simulink model "Starting_v2"  (R2020b)
settings: Solver=ode45  StartTime=0.0  StopTime=0.6  MaxStep=1e-6  RelTol=1e-3
InitFcn:
  | Parameters
undefined symbols (not defined in the file): C_LUT, E_in, fsw, Io_target, ki, kp, L_in, R_in, R_LUT, R_sd, V_OC_LUT, V_soc_0
libraries: simulink x3
settings Model: Creator=sandr  LastModifiedBy=sandr

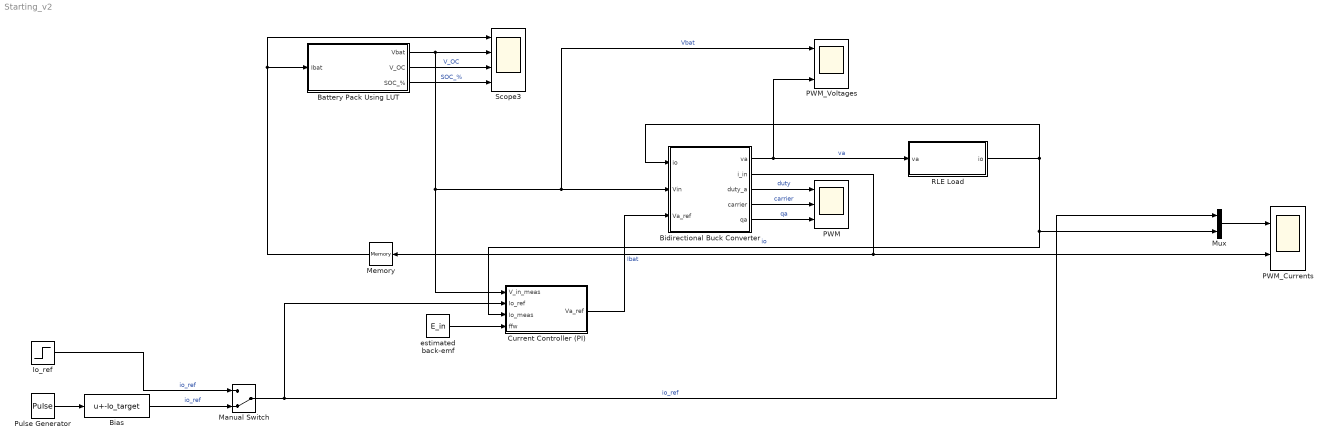
== system Starting_v2 ==
  Battery Pack Using LUT : Subsystem  mask(Battery Pack Model){Cq=C_LUT, Rsd=R_sd, V_SOC_0=V_soc_0, data=V_OC_LUT, R0=R_LUT}
      mask prompts: Cq "Battery Capacity - Cq (As)"; Rsd "Internal Discharging Resistance - Rsd (Ohm)"; V_SOC_0 "Initial V_SOC_0"; data "V_OC from LUT"; R0 "Series Resistance - R0 (Ohm)"
      mask help: This block implements the model of a battery pack.
      mask Help: Author: Sandro Rubino
  Bias : Bias  Bias=-Io_target
  Bidirectional Buck Converter : Subsystem  mask(Bidirectional Buck Converter){fsw=fsw}
      mask prompts: fsw "Switching Frequency - fsw (Hz)"
  Current Controller (PI) : Subsystem  mask(Current Controller (PI Regulator)){kp=kp, ki=ki}
      mask prompts: kp "Proportional Gain - kp (V/A)"; ki "Integral Gain - ki (V/A/s)"
      mask help: This block implments a PI regulator/controller for current control.
  Io_ref : Step  Time=0.3  After=800  SampleTime=0
  Manual Switch : ManualSwitch  CurrentSetting=0
  Memory : Memory
  Mux : Mux  Inputs=2
  PWM : Scope  NumInputPorts=3
  PWM_Currents : Scope  NumInputPorts=2
  PWM_Voltages : Scope  NumInputPorts=3
  Pulse Generator : DiscretePulseGenerator  PulseType=Time based  Amplitude=2*Io_target  Period=0.2  PulseWidth=50
  RLE Load : Subsystem  mask(RLE Load){R=R_in, L=L_in, E=E_in}
      mask prompts: R "Resistance - R (ohm)"; L "Inductance - L (H)"; E "Back-emf - E (V)"
  Scope3 : Scope  NumInputPorts=4
  estimated back-emf : Constant  Value=E_in
  wires:
  Battery Pack Using LUT/3(SOC_%) -> Scope3/4  "SOC_%"
  Battery Pack Using LUT/2(V_OC) -> Scope3/3  "V_OC"
  Battery Pack Using LUT/1(Vbat) -> Current Controller (PI)/1(V_in_meas), PWM_Voltages/1, Bidirectional Buck Converter/2(Vin), Scope3/2  "Vbat"
  Bidirectional Buck Converter/1(va) -> PWM_Voltages/3, RLE Load/1(va)  "va"
  RLE Load/1(io) -> Current Controller (PI)/3(Io_meas), Mux/2, Bidirectional Buck Converter/1(io)  "io"
  Bidirectional Buck Converter/2(i_in) -> Memory/1, PWM_Currents/2  "Ibat"
  Memory/1 -> Battery Pack Using LUT/1(Ibat), Scope3/1
  Bidirectional Buck Converter/3(duty_a) -> PWM/1  "duty"
  Bidirectional Buck Converter/4(carrier) -> PWM/2  "carrier"
  Bidirectional Buck Converter/5(qa) -> PWM/3  "qa"
  Mux/1 -> PWM_Currents/1
  Current Controller (PI)/1(Va_ref) -> Bidirectional Buck Converter/3(Va_ref)
  Manual Switch/1 -> Current Controller (PI)/2(Io_ref), Mux/1  "io_ref"
  Pulse Generator/1 -> Bias/1
  Bias/1 -> Manual Switch/2  "io_ref"
  Io_ref/1 -> Manual Switch/1  "io_ref"
  estimated back-emf/1 -> Current Controller (PI)/4(ffw)

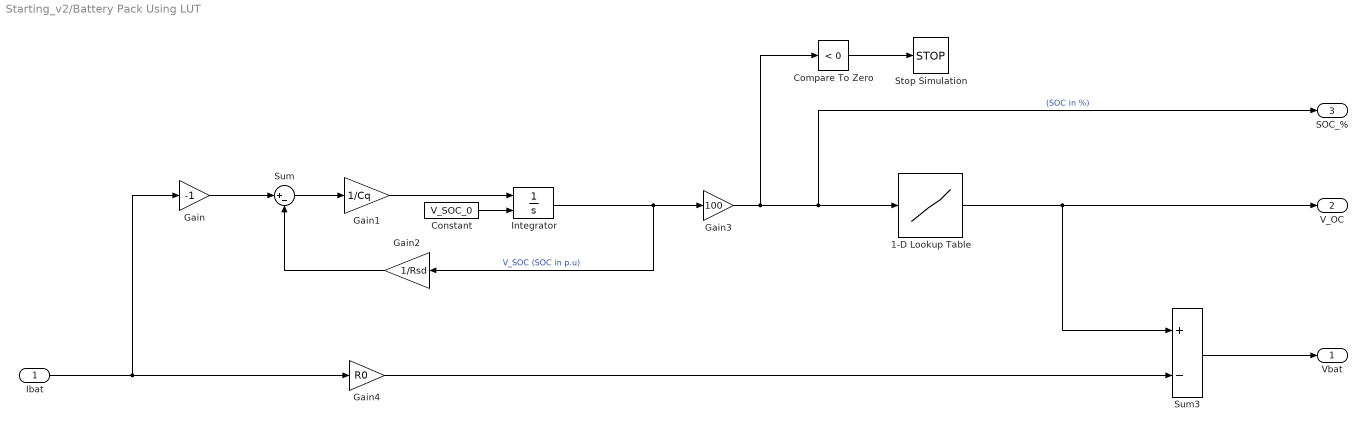
== system Starting_v2/Battery Pack Using LUT ==
  Ibat : Inport
  1-D Lookup Table : Lookup_n-D  NumberOfTableDimensions=1  BreakpointsForDimension1=0:1:100  Table=data  InternalRulePriority=Speed  RndMeth=Simplest  InputSameDT=on
  Compare To Zero : simulink/Logic and Bit Operations/Compare To Zero  relop=<  OutDataTypeStr=boolean
  Constant : Constant  Value=V_SOC_0
  Gain : Gain  Gain=-1
  Gain1 : Gain  Gain=1/Cq
  Gain2 : Gain  Gain=1/Rsd
  Gain3 : Gain  Gain=100
  Gain4 : Gain  Gain=R0
  Integrator : Integrator  InitialConditionSource=external
  Stop Simulation : Stop
  Sum : Sum  Inputs=|+-
  Sum3 : Sum  Inputs=+-
  Vbat : Outport
  V_OC : Outport  Port=2
  SOC_% : Outport  Port=3
  wires:
  Sum/1 -> Gain1/1
  Sum3/1 -> Vbat/1
  Gain3/1 -> Compare To Zero/1, 1-D Lookup Table/1, SOC_%/1  "(SOC in %)"
  Constant/1 -> Integrator/2
  Gain1/1 -> Integrator/1
  Integrator/1 -> Gain3/1, Gain2/1  "V_SOC (SOC in p.u)"
  Gain/1 -> Sum/1
  Gain4/1 -> Sum3/2
  Gain2/1 -> Sum/2
  Ibat/1 -> Gain4/1, Gain/1
  Compare To Zero/1 -> Stop Simulation/1
  1-D Lookup Table/1 -> Sum3/1, V_OC/1

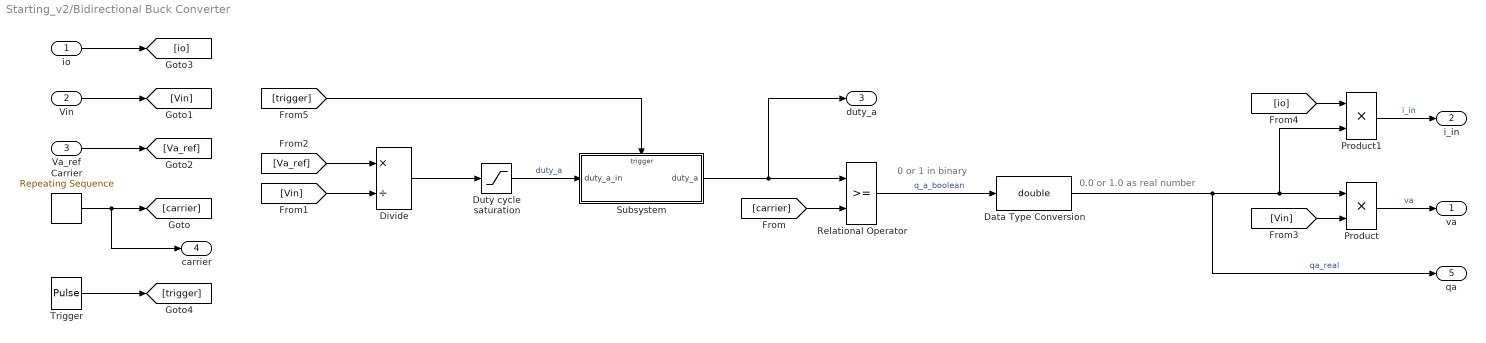
== system Starting_v2/Bidirectional Buck Converter ==
  note: 0.0 or 1.0 as real number
  note: 0 or 1 in binary
  io : Inport
  Vin : Inport  Port=2
  Va_ref : Inport  Port=3
  Carrier : simulink/Sources/Repeating Sequence  rep_seq_t=[0 0.5/fsw 1/fsw]  rep_seq_y=[0 1 0]
  Data Type Conversion : DataTypeConversion  OutDataTypeStr=double
  Divide : Product  Inputs=*/
  Duty cycle saturation : Saturate  UpperLimit=1  LowerLimit=0
  Product : Product
  Product1 : Product
  Relational Operator : RelationalOperator  OutDataTypeStr=boolean  RndMeth=Simplest
  Subsystem : Subsystem
  Trigger : DiscretePulseGenerator  PulseType=Time based  Period=1/fsw  PulseWidth=50
  va : Outport
  i_in : Outport  Port=2
  duty_a : Outport  Port=3
  carrier : Outport  Port=4
  qa : Outport  Port=5
  wires:
  Carrier/1 -> carrier/1, [carrier]
  Vin/1 -> [Vin]
  Va_ref/1 -> [Va_ref]
  [Va_ref] -> Divide/1
  [Vin] -> Divide/2
  [Vin] -> Product/2
  Product/1 -> va/1  "va"
  io/1 -> [io]
  [io] -> Product1/1
  Product1/1 -> i_in/1  "i_in"
  Trigger/1 -> [trigger]
  [carrier] -> Relational Operator/2
  Data Type Conversion/1 -> qa/1, Product/1, Product1/2  "qa_real"
  Relational Operator/1 -> Data Type Conversion/1  "q_a_boolean"
  Divide/1 -> Duty cycle saturation/1
  Subsystem/1(duty_a) -> duty_a/1, Relational Operator/1
  [trigger] -> Subsystem/Trigger
  Duty cycle saturation/1 -> Subsystem/1(duty_a_in)  "duty_a"

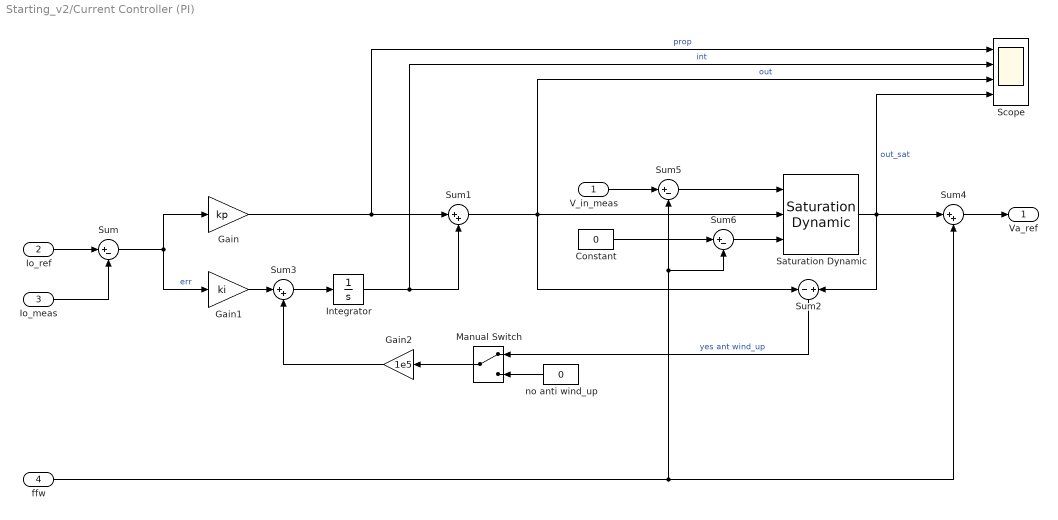
== system Starting_v2/Current Controller (PI) ==
  V_in_meas : Inport
  Io_ref : Inport  Port=2
  Io_meas : Inport  Port=3
  ffw : Inport  Port=4
  Constant : Constant  Value=0
  Gain : Gain  Gain=kp
  Gain1 : Gain  Gain=ki
  Gain2 : Gain  Gain=1e5
  Integrator : Integrator
  Manual Switch : ManualSwitch
  Saturation Dynamic : simulink/Discontinuities/Saturation Dynamic  OutMin=[]  OutMax=[]  OutDataTypeStr=Inherit: Same as second input  OutDataType=fixdt(1, 16)  OutScaling=2^-10  DoSatur=off
  Scope : Scope  NumInputPorts=4
  Sum : Sum  Inputs=|+-
  Sum1 : Sum  Inputs=|++
  Sum2 : Sum  Inputs=-+
  Sum3 : Sum  Inputs=|++
  Sum4 : Sum  Inputs=|++
  Sum5 : Sum  Inputs=|+-
  Sum6 : Sum  Inputs=|+-
  no anti wind_up : Constant  Value=0
  Va_ref : Outport
  wires:
  Io_ref/1 -> Sum/1
  Io_meas/1 -> Sum/2
  Sum/1 -> Gain1/1, Gain/1  "err"
  Gain1/1 -> Sum3/1
  Gain/1 -> Scope/1, Sum1/1  "prop"
  Integrator/1 -> Scope/2, Sum1/2  "int"
  Sum1/1 -> Sum2/1, Saturation Dynamic/2, Scope/3  "out"
  V_in_meas/1 -> Sum5/1
  Constant/1 -> Sum6/1
  Saturation Dynamic/1 -> Sum4/1, Sum2/2, Scope/4  "out_sat"
  Sum2/1 -> Manual Switch/1  "yes ant wind_up"
  Sum3/1 -> Integrator/1
  Gain2/1 -> Sum3/2
  Manual Switch/1 -> Gain2/1
  no anti wind_up/1 -> Manual Switch/2
  Sum4/1 -> Va_ref/1
  ffw/1 -> Sum6/2, Sum5/2, Sum4/2
  Sum6/1 -> Saturation Dynamic/3
  Sum5/1 -> Saturation Dynamic/1

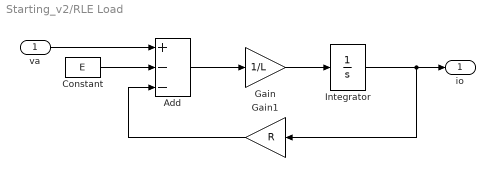
== system Starting_v2/RLE Load ==
  va : Inport
  Add : Sum  Inputs=+--
  Constant : Constant  Value=E
  Gain : Gain  Gain=1/L
  Gain1 : Gain  Gain=R
  Integrator : Integrator
  io : Outport
  wires:
  va/1 -> Add/1
  Constant/1 -> Add/2
  Add/1 -> Gain/1
  Gain1/1 -> Add/3
  Gain/1 -> Integrator/1
  Integrator/1 -> Gain1/1, io/1

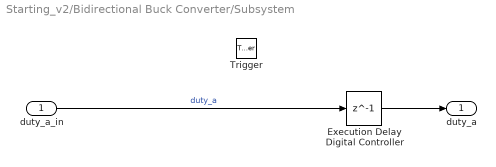
== system Starting_v2/Bidirectional Buck Converter/Subsystem ==
  duty_a_in : Inport
  Trigger : TriggerPort  VariantControl=Variant  PortDimensions=1
  Execution Delay Digital Controller : Delay  DelayLength=1  InitialCondition=0
  duty_a : Outport  InitialOutput=[1]
  wires:
  duty_a_in/1 -> Execution Delay Digital Controller/1  "duty_a"
  Execution Delay Digital Controller/1 -> duty_a/1
